simulink model "modifiaud1"  (R2015b)
settings: Solver=FixedStepDiscrete  SolverMode=SingleTasking  StartTime=0.0  StopTime=300  RelTol=1e-3
libraries: xbsIndex_r4 x85, simulink x2
settings Model: Creator=spiro user  LastModifiedBy=HANI
settings DataIOCC: SaveFormat=Array
settings DebuggingCC: UnderspecifiedInitializationDetection=Classic  MergeDetectMultiDrivingBlocksExec=none  SolverPrmCheckMsg=warning  StateNameClashWarn=warning
settings HardwareCC: ProdBitPerPointer=32  ProdLargestAtomicFloat=None  ProdIntDivRoundTo=Undefined  ProdEndianess=Unspecified  ProdWordSize=32  ProdHWDeviceType=32-bit Generic
settings GRTTargetCC: GeneratePreprocessorConditionals=Disable all
settings ConfigComp: CovModelRefEnable=Off

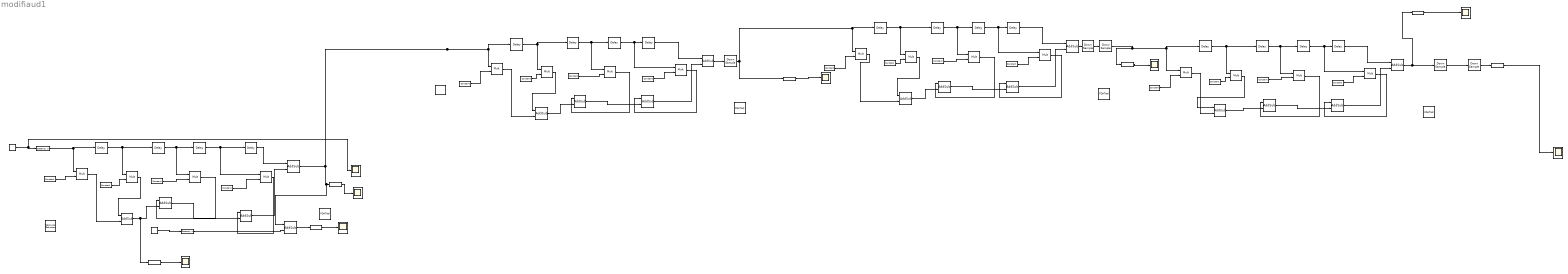
== system modifiaud1 ==
  " System Generator" : xbsIndex_r4/ System Generator  Tag=genX  xilinxfamily=artix7  part=xc7a200t  speed=-3  package=fbg676  synthesis_tool=XST  clock_wrapper=Clock Enables  directory=D:/Ramkumar. R- xsg/blind/v-code  proj_type=Project Navigator  Synth_file=XST Defaults  Impl_file=ISE Defaults  testbench=off  simulink_period=1  sysclk_period=20  dcm_input_clock_period=10  incr_netlist=off  trim_vbits=Everywhere in SubSystem  dbl_ovrd=According to Block Masks  core_generation=According to Block Masks  run_coregen=off  deprecated_control=off  eval_field=0  block_type=sysgen
  AddSub{1..4,9..16,24..27} (16 alike) : xbsIndex_r4/AddSub  mode=Addition  use_carryin=off  use_carryout=off  en=off  latency=0  precision=Full  arith_type=Unsigned  n_bits=16  bin_pt=14  quantization=Truncate  overflow=Wrap  dbl_ovrd=off  use_behavioral_HDL=off  hw_selection=Fabric  pipelined=off  block_type=addsub
      AddSub1 settings: xl_area=[10 0 0 18 0 0 0]
      AddSub10 settings: xl_area=[9 0 0 17 0 0 0]
      AddSub11 settings: xl_area=[9 0 0 16 0 0 0]
      AddSub12 settings: xl_area=[11 0 0 20 0 0 0]
      AddSub13 settings: xl_area=[9 0 0 17 0 0 0]
      AddSub14 settings: xl_area=[9 0 0 16 0 0 0]
      AddSub15 settings: xl_area=[11 0 0 21 0 0 0]
      AddSub16 settings: xl_area=[10 0 0 18 0 0 0]
      AddSub2 settings: xl_area=[9 0 0 17 0 0 0]
      AddSub24 settings: xl_area=[9 0 0 17 0 0 0]
      AddSub25 settings: xl_area=[9 0 0 16 0 0 0]
      AddSub26 settings: xl_area=[12 0 0 22 0 0 0]
      AddSub27 settings: xl_area=[10 0 0 18 0 0 0]
      AddSub3 settings: xl_area=[9 0 0 16 0 0 0]
      AddSub4 settings: xl_area=[10 0 0 19 0 0 0]
      AddSub9 settings: xl_area=[10 0 0 18 0 0 0]
  AddSub29 : xbsIndex_r4/AddSub  mode=Subtraction  use_carryin=off  use_carryout=off  en=off  latency=0  precision=Full  arith_type=Unsigned  n_bits=16  bin_pt=14  quantization=Truncate  overflow=Wrap  dbl_ovrd=off  use_behavioral_HDL=off  hw_selection=Fabric  pipelined=off  block_type=addsub
      settings: xl_area=[11 0 0 20 0 0 0]
  Band-Limited White Noise1 : simulink/Sources/Band-Limited White Noise  Cov=[0.1]  Ts=0.1  seed=[23341]
  Band-Limited White Noise2 : simulink/Sources/Band-Limited White Noise  Cov=[0.1]  Ts=0.1  seed=[23341]
  Constant1 : xbsIndex_r4/Constant  const=-0.052471954387914473  gui_display_data_type=Fixed-point  arith_type=Signed (2's comp)  n_bits=16  bin_pt=14  preci_type=Double  exp_width=8  frac_width=24  explicit_period=on  period=1  equ=P=C  opselect=C  inp2=PCIN>>17  opr=+  inp1=P  carry=CIN  dbl_ovrd=off  block_type=constant
  Constant10 : xbsIndex_r4/Constant  const=0.31017558451132293  gui_display_data_type=Fixed-point  arith_type=Signed (2's comp)  n_bits=16  bin_pt=14  preci_type=Double  exp_width=8  frac_width=24  explicit_period=on  period=1  equ=P=C  opselect=C  inp2=PCIN>>17  opr=+  inp1=P  carry=CIN  dbl_ovrd=off  block_type=constant
  Constant11 : xbsIndex_r4/Constant  const=0.0524719543879145  gui_display_data_type=Fixed-point  arith_type=Signed (2's comp)  n_bits=16  bin_pt=14  preci_type=Double  exp_width=8  frac_width=24  explicit_period=on  period=1  equ=P=C  opselect=C  inp2=PCIN>>17  opr=+  inp1=P  carry=CIN  dbl_ovrd=off  block_type=constant
  Constant12 : xbsIndex_r4/Constant  const=0.44427464606198364  gui_display_data_type=Fixed-point  arith_type=Signed (2's comp)  n_bits=16  bin_pt=14  preci_type=Double  exp_width=8  frac_width=24  explicit_period=off  period=1  equ=P=C  opselect=C  inp2=PCIN>>17  opr=+  inp1=P  carry=CIN  dbl_ovrd=off  block_type=constant
  Constant13 : xbsIndex_r4/Constant  const=0.0524719543879145  gui_display_data_type=Fixed-point  arith_type=Signed (2's comp)  n_bits=16  bin_pt=14  preci_type=Double  exp_width=8  frac_width=24  explicit_period=on  period=1  equ=P=C  opselect=C  inp2=PCIN>>17  opr=+  inp1=P  carry=CIN  dbl_ovrd=off  block_type=constant
  Constant14 : xbsIndex_r4/Constant  const=0.0524719543879145  gui_display_data_type=Fixed-point  arith_type=Signed (2's comp)  n_bits=16  bin_pt=14  preci_type=Double  exp_width=8  frac_width=24  explicit_period=on  period=1  equ=P=C  opselect=C  inp2=PCIN>>17  opr=+  inp1=P  carry=CIN  dbl_ovrd=off  block_type=constant
  Constant15 : xbsIndex_r4/Constant  const=0.31017558451132293  gui_display_data_type=Fixed-point  arith_type=Signed (2's comp)  n_bits=16  bin_pt=14  preci_type=Double  exp_width=8  frac_width=24  explicit_period=off  period=1  equ=P=C  opselect=C  inp2=PCIN>>17  opr=+  inp1=P  carry=CIN  dbl_ovrd=off  block_type=constant
  Constant2 : xbsIndex_r4/Constant  const=-0.31017558451132293  gui_display_data_type=Fixed-point  arith_type=Signed (2's comp)  n_bits=16  bin_pt=14  preci_type=Double  exp_width=8  frac_width=24  explicit_period=on  period=1  equ=P=C  opselect=C  inp2=PCIN>>17  opr=+  inp1=P  carry=CIN  dbl_ovrd=off  block_type=constant
  Constant20 : xbsIndex_r4/Constant  const=0.31017558451132293  gui_display_data_type=Fixed-point  arith_type=Signed (2's comp)  n_bits=16  bin_pt=14  preci_type=Double  exp_width=8  frac_width=24  explicit_period=on  period=1  equ=P=C  opselect=C  inp2=PCIN>>17  opr=+  inp1=P  carry=CIN  dbl_ovrd=off  block_type=constant
  Constant21 : xbsIndex_r4/Constant  const=0.44427464606198364  gui_display_data_type=Fixed-point  arith_type=Signed (2's comp)  n_bits=16  bin_pt=14  preci_type=Double  exp_width=8  frac_width=24  explicit_period=off  period=1  equ=P=C  opselect=C  inp2=PCIN>>17  opr=+  inp1=P  carry=CIN  dbl_ovrd=off  block_type=constant
  Constant22 : xbsIndex_r4/Constant  const=0.31017558451132293  gui_display_data_type=Fixed-point  arith_type=Signed (2's comp)  n_bits=16  bin_pt=14  preci_type=Double  exp_width=8  frac_width=24  explicit_period=off  period=1  equ=P=C  opselect=C  inp2=PCIN>>17  opr=+  inp1=P  carry=CIN  dbl_ovrd=off  block_type=constant
  Constant3 : xbsIndex_r4/Constant  const=-0.31017558451132293  gui_display_data_type=Fixed-point  arith_type=Signed (2's comp)  n_bits=16  bin_pt=14  preci_type=Double  exp_width=8  frac_width=24  explicit_period=on  period=1  equ=P=C  opselect=C  inp2=PCIN>>17  opr=+  inp1=P  carry=CIN  dbl_ovrd=off  block_type=constant
  Constant32 : xbsIndex_r4/Constant  const=0.31017558451132293  gui_display_data_type=Fixed-point  arith_type=Signed (2's comp)  n_bits=16  bin_pt=14  preci_type=Double  exp_width=8  frac_width=24  explicit_period=on  period=1  equ=P=C  opselect=C  inp2=PCIN>>17  opr=+  inp1=P  carry=CIN  dbl_ovrd=off  block_type=constant
  Constant34 : xbsIndex_r4/Constant  const=0.55572535393801636  gui_display_data_type=Fixed-point  arith_type=Signed (2's comp)  n_bits=16  bin_pt=14  preci_type=Double  exp_width=8  frac_width=24  explicit_period=on  period=1  equ=P=C  opselect=C  inp2=PCIN>>17  opr=+  inp1=P  carry=CIN  dbl_ovrd=off  block_type=constant
  Constant8 : xbsIndex_r4/Constant  const=0.31017558451132293  gui_display_data_type=Fixed-point  arith_type=Signed (2's comp)  n_bits=16  bin_pt=14  preci_type=Double  exp_width=8  frac_width=24  explicit_period=off  period=1  equ=P=C  opselect=C  inp2=PCIN>>17  opr=+  inp1=P  carry=CIN  dbl_ovrd=off  block_type=constant
  Constant9 : xbsIndex_r4/Constant  const=0.44427464606198364  gui_display_data_type=Fixed-point  arith_type=Signed (2's comp)  n_bits=16  bin_pt=14  preci_type=Double  exp_width=8  frac_width=24  explicit_period=off  period=1  equ=P=C  opselect=C  inp2=PCIN>>17  opr=+  inp1=P  carry=CIN  dbl_ovrd=off  block_type=constant
  Delay{,2..3,8..15,20..23,32} (16 alike) : xbsIndex_r4/Delay  rst=off  infoeditControl=Selection of Reset will increase slice count due to use of real FFs and instead of SRLs  en=off  latency=1  dbl_ovrd=off  reg_retiming=off  block_type=delay
  Down Sample1 : xbsIndex_r4/Down Sample  sample_ratio=2  sample_phase="Last Value of Frame  (most efficient)"  en=off  latency=1  dbl_ovrd=off  block_type=dsamp
  Down Sample10 : xbsIndex_r4/Down Sample  sample_ratio=3  sample_phase="Last Value of Frame  (most efficient)"  en=off  latency=1  dbl_ovrd=off  block_type=dsamp
  Down Sample2 : xbsIndex_r4/Down Sample  sample_ratio=2  sample_phase="Last Value of Frame  (most efficient)"  en=off  latency=1  dbl_ovrd=off  block_type=dsamp
  Down Sample4 : xbsIndex_r4/Down Sample  sample_ratio=5  sample_phase="Last Value of Frame  (most efficient)"  en=off  latency=1  dbl_ovrd=off  block_type=dsamp
  Down Sample7 : xbsIndex_r4/Down Sample  sample_ratio=4  sample_phase="Last Value of Frame  (most efficient)"  en=off  latency=1  dbl_ovrd=off  block_type=dsamp
  FDATool{,2..3,6} (4 alike) : xbsIndex_r4/FDATool  block_type=fdatool
      settings: infoedit=FDATool
  Gateway In : xbsIndex_r4/Gateway In  gui_display_data_type=Fixed-point  arith_type="Signed  (2's comp)"  n_bits=16  bin_pt=14  preci_type=Double  exp_width=8  frac_width=24  quantization=Truncate  overflow=Wrap  period=1  dbl_ovrd=off  timing_constraint=None  locs_specified=off  LOCs={}  UseAsADC=off  ADCChannel='1'  inherit_from_input=off  hdl_port=on  block_type=gatewayin
  Gateway In1 : xbsIndex_r4/Gateway In  gui_display_data_type=Fixed-point  arith_type="Signed  (2's comp)"  n_bits=16  bin_pt=14  preci_type=Double  exp_width=8  frac_width=24  quantization=Truncate  overflow=Wrap  period=1  dbl_ovrd=off  timing_constraint=None  locs_specified=off  LOCs={}  UseAsADC=off  ADCChannel='1'  inherit_from_input=off  hdl_port=on  block_type=gatewayin
  Gateway Out{,1..3,5,8,11} (7 alike) : xbsIndex_r4/Gateway Out  inherit_from_input=off  hdl_port=on  timing_constraint=None  locs_specified=off  LOCs={}  UseAsDAC=off  DACChannel='1'  block_type=gatewayout
  Mult{,1..3,8..15,20..23} (16 alike) : xbsIndex_r4/Mult  precision=User Defined  arith_type="Signed  (2's comp)"  n_bits=16  bin_pt=14  quantization=Truncate  overflow=Wrap  en=off  latency=3  dbl_ovrd=off  use_behavioral_HDL=off  opt=Speed  use_embedded=on  optimum_pipeline=off  pipeline=on  use_rpm=on  placement_style=Triangular  block_type=mult
  Resource Estimator : xbsIndex_r4/Resource Estimator  Tag=resEstTag  Slices=0  FFs=0  BRAMs=0  LUTs=0  IOBs=0  EBMs=0  TBUFs=0  xl_use_estimator_area=off  est_options=Estimate  block_type=resource_estimator
      settings: AttributesFormatString=Resource\nEstimator
  Time Scope{,1..3,5,8..9,12} (8 alike) : Scope
  wires:
  Delay3/1 -> Mult/1, Delay2/1
  Mult2/1 -> AddSub3/2
  Mult1/1 -> AddSub3/1
  AddSub3/1 -> Gateway Out11/1, AddSub2/2
  Mult/1 -> AddSub2/1
  Delay2/1 -> Delay32/1, Mult3/1
  Band-Limited White Noise2/1 -> Time Scope/1, Gateway In/1
  Gateway Out/1 -> Time Scope1/1
  Constant11/1 -> Mult10/2
  Delay11/1 -> Mult8/1, Delay10/1
  Mult10/1 -> AddSub11/2
  AddSub4/1 -> AddSub29/1, Gateway Out/1, Delay8/1, Mult10/1
  Constant10/1 -> Mult9/2
  Mult9/1 -> AddSub11/1
  Constant9/1 -> Mult8/2
  AddSub11/1 -> AddSub10/2
  Mult8/1 -> AddSub10/1
  Constant8/1 -> Mult11/2
  Delay10/1 -> Mult11/1, Delay9/1
  AddSub10/1 -> AddSub9/2
  Mult11/1 -> AddSub9/1
  AddSub9/1 -> AddSub12/2
  Gateway Out2/1 -> Time Scope3/1
  Constant13/1 -> Mult12/2
  Mult12/1 -> AddSub14/2
  Constant32/1 -> Mult15/2
  Mult15/1 -> AddSub14/1
  Constant12/1 -> Mult14/2
  AddSub14/1 -> AddSub13/2
  Mult14/1 -> AddSub13/1
  Constant15/1 -> Mult13/2
  AddSub13/1 -> AddSub16/2
  Mult13/1 -> AddSub16/1
  AddSub16/1 -> AddSub15/2
  Delay15/1 -> AddSub15/1
  Gateway Out3/1 -> Time Scope5/1
  AddSub12/1 -> Down Sample2/1
  Constant14/1 -> Mult20/2
  Delay21/1 -> Mult22/1, Delay20/1
  Mult20/1 -> AddSub25/2
  Delay22/1 -> Mult23/1, Delay21/1
  Constant20/1 -> Mult23/2
  Mult23/1 -> AddSub25/1
  Constant21/1 -> Mult22/2
  Mult22/1 -> AddSub24/1
  Constant22/1 -> Mult21/2
  Delay20/1 -> Mult21/1, Delay23/1
  Mult21/1 -> AddSub27/1
  Delay23/1 -> AddSub26/1
  AddSub15/1 -> Down Sample1/1
  Band-Limited White Noise1/1 -> Gateway In1/1
  AddSub29/1 -> Gateway Out8/1
  Gateway Out8/1 -> Time Scope9/1
  Delay14/1 -> Mult15/1, Delay13/1
  Delay13/1 -> Mult14/1, Delay12/1
  Delay12/1 -> Mult13/1, Delay15/1
  AddSub2/1 -> AddSub1/2
  Mult3/1 -> AddSub1/1
  AddSub1/1 -> AddSub4/2
  Down Sample2/1 -> Gateway Out2/1, Delay14/1, Mult12/1
  Gateway Out5/1 -> Time Scope8/1
  Down Sample10/1 -> Gateway Out5/1
  AddSub26/1 -> Gateway Out1/1, Down Sample7/1
  Gateway In1/1 -> AddSub29/2
  Down Sample1/1 -> Down Sample4/1
  AddSub27/1 -> AddSub26/2
  AddSub24/1 -> AddSub27/2
  AddSub25/1 -> AddSub24/2
  Delay32/1 -> AddSub4/1
  Delay/1 -> Delay3/1, Mult1/1
  Gateway In/1 -> Delay/1, Mult2/1
  Delay8/1 -> Delay11/1, Mult9/1
  Delay9/1 -> AddSub12/1
  Constant1/1 -> Mult2/2
  Constant34/1 -> Mult/2
  Constant2/1 -> Mult3/2
  Constant3/1 -> Mult1/2
  Gateway Out11/1 -> Time Scope12/1
  Down Sample4/1 -> Gateway Out3/1, Delay22/1, Mult20/1
  Down Sample7/1 -> Down Sample10/1
  Gateway Out1/1 -> Time Scope2/1
